simulink model "inverse_dynamics_1dof_robust"  (R2023b)
settings: Solver=VariableStepAuto  StartTime=0.0  StopTime=Tend_slk  RelTol=1e-3
values from neighbouring files (symbols this model uses):
  Kd = 0.01333    [PI_inverse.mat]    (also in main_inverse_1dof.m)
  Kp = 6.221e-06    [PI_inverse.mat]    (also in main_inverse_1dof.m = 3.111e-06)
  param = [Ixx;Iyy;Izz;l;k;b;m]    [EKF_main_inverse_1dof.m]    (also in EKF_main_inverse_1dof_robust.m = [Ixx;Iyy;Izz;l;k1;k2;k3;k4;b;m]; main_inverse_1dof.m)
  Ts_slk = 0.01    [EKF_main_inverse_1dof.m]    (also in EKF_main_inverse_1dof_robust.m; main_inverse_1dof.m)
  x0 = [1;1;1;0;0;0]*0.01    [EKF_main_inverse_1dof.m]    (also in EKF_main_inverse_1dof_robust.m; main_inverse_1dof.m = [0;0])
undefined symbols (not defined in the file or in its folder): x_eq
settings Model: Creator=asus  LastModifiedBy=asus
settings OptimizationCC: ReuseModelBlockBuffer=off

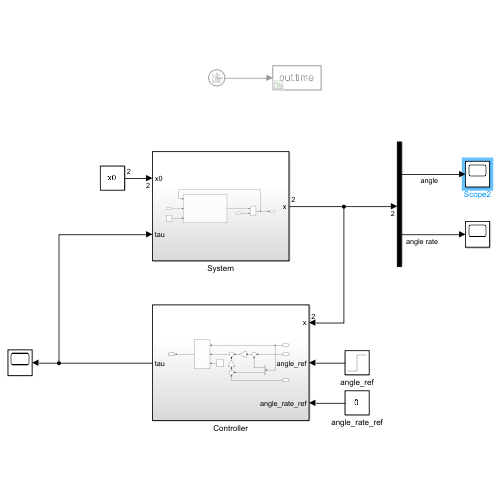
[thumbnail: Simulink's stored preview of the top-level diagram]
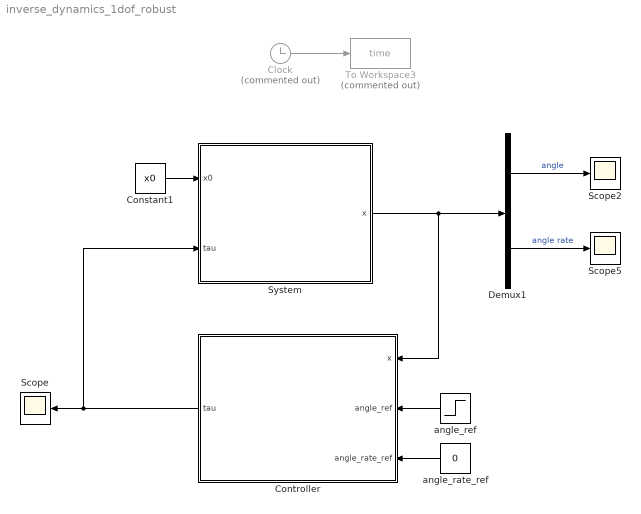
== system inverse_dynamics_1dof_robust ==
  Clock : Clock  Commented=on
  Constant1 : Constant  Value=x0
  Controller : Subsystem
  Demux1 : Demux  Outputs=2
  Scope : Scope
  Scope2 : Scope
  Scope5 : Scope
  System : Subsystem
  To Workspace3 : ToWorkspace  Commented=on  VariableName=time  SampleTime=Ts_slk
      settings: Save2DSignal=2-D array (concatenate along first dimension)
  angle_rate_ref : Constant  Value=0
  angle_ref : Step  Time=0  After=30*pi/180  SampleTime=Ts_slk
  wires:
  Clock/1 -> To Workspace3/1
  System/1(x) -> Controller/1(x), Demux1/1
  Demux1/2 -> Scope5/1  "angle rate"
  Demux1/1 -> Scope2/1  "angle"
  Controller/1(tau) -> Scope/1, System/2("tau ")
  angle_ref/1 -> Controller/2(angle_ref)
  angle_rate_ref/1 -> Controller/3(angle_rate_ref)
  Constant1/1 -> System/1(x0)

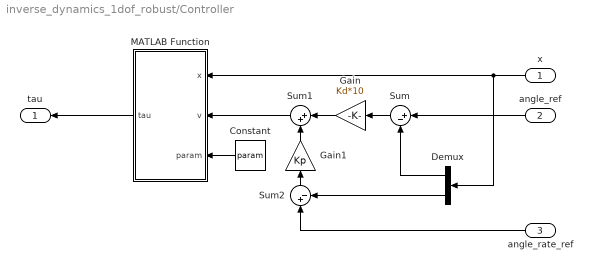
== system inverse_dynamics_1dof_robust/Controller ==
  x : Inport
  angle_ref : Inport  Port=2
  angle_rate_ref : Inport  Port=3
  Constant : Constant  Value=param
  Demux : Demux  Outputs=2
  Gain : Gain  Gain=Kd*10
  Gain1 : Gain  Gain=Kp
  MATLAB Function : MATLAB Function  TreatAsAtomicUnit=on
  Sum : Sum  Inputs=|+-
  Sum1 : Sum  Inputs=|++
  Sum2 : Sum  Inputs=|+-
  tau : Outport
  wires:
  Constant/1 -> MATLAB Function/3(param)
  x/1 -> Demux/1, MATLAB Function/1(x)
  MATLAB Function/1(tau) -> tau/1
  angle_ref/1 -> Sum/1
  angle_rate_ref/1 -> Sum2/1
  Sum1/1 -> MATLAB Function/2(v)
  Gain/1 -> Sum1/1
  Gain1/1 -> Sum1/2
  Sum2/1 -> Gain1/1
  Sum/1 -> Gain/1
  Demux/1 -> Sum/2
  Demux/2 -> Sum2/2

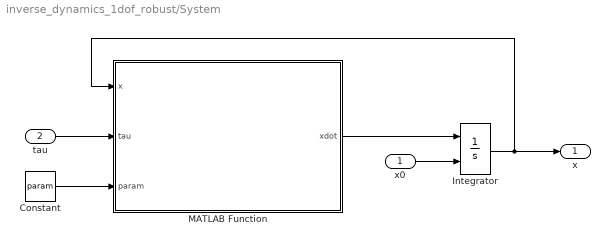
== system inverse_dynamics_1dof_robust/System ==
  x0 : Inport
  "tau " : Inport  Port=2
  Constant : Constant  Value=param
  Integrator : Integrator  InitialConditionSource=external  InitialCondition=x_eq
  MATLAB Function : MATLAB Function  TreatAsAtomicUnit=on
  x : Outport
  wires:
  Integrator/1 -> MATLAB Function/1(x), x/1
  MATLAB Function/1(xdot) -> Integrator/1
  "tau "/1 -> MATLAB Function/2(tau)
  Constant/1 -> MATLAB Function/3(param)
  x0/1 -> Integrator/2

== matlab function inverse_dynamics_1dof_robust/System/MATLAB Function ==
  data: x input; tau input; xdot output; param input
function xdot=quadcopter(x,tau,param)
% Inputs:
%           x       (model state)
%           tau     (torque)           
%           param   (model parameters)
%
% Outputs:  x_dot  (derivative of the state with respect to time)

% Parameters
g        =       9.81;           %  gravity acceleration (m/s^2)
Ixx      =       param(1,1);     %  moment of inertia 

% States
phi         =       x(1,1);      %  roll angle (rad)
phi_dot     =       x(2,1);      %  roll rate (rad/s)


cph         =       cos(phi);
sph         =       sin(phi);

% State space model
xdot        = zeros(2,1);
xdot(1,1)   = phi_dot;
xdot(2,1)   = tau/Ixx;

== matlab function inverse_dynamics_1dof_robust/Controller/MATLAB Function ==
  data: x input; v input; tau output; param input
function tau = fcn(x,v,param)
% Inputs:
%           x       (model state)
%           v       (new input to the feedback system)           
%           param   (model parameters)
%
% Outputs:  tau  (torque)

% Parameters
g        =       9.81;           %  gravity acceleration (m/s^2)
Ixx      =       param(1,1);     %  moment of inertia 

% States
phi         =       x(1,1);      %  roll angle (rad)
phi_dot     =       x(2,1);      %  roll rate (rad/s)


cph         =       cos(phi);
sph         =       sin(phi);


% Inertia matrix
J= Ixx;

% control law
tau = 0;
tau = J*v;
